simulink model "NCO_lfm_test"  (R2019b)
settings: Solver=FixedStepDiscrete  StartTime=0.0  StopTime=stoptime  RelTol=1e-3
InitFcn:
  | model_init
values from neighbouring files (symbols this model uses):
  chirp_dur_samp = fs*chirp_dur    (= 6400)    [model_init.m]
  end_inc = floor(f1*2^N / fs)    [model_init.m]
  start_inc = floor(f0*2^N / fs)    [model_init.m]
  Ts = 1/fs    (= 7.8125e-09)    [model_init.m]
libraries: hdlsllib x1, dsphdlsigops x1, dspsrcs4 x1
settings Model: DataTypeOverride=Off  Creator=tmealey  LastModifiedBy=ajtro
settings DataIOCC: SaveOutput=off  SignalLogging=off  DSMLogging=off  SaveTime=off  ReturnWorkspaceOutputs=off
settings OptimizationCC: BlockReduction=off  ConditionallyExecuteInputs=off  DefaultParameterBehavior=Inlined
settings DebuggingCC: AlgebraicLoopMsg=error  SingleTaskRateTransMsg=error
settings HardwareCC: ProdBitPerPointer=32  ProdBitPerSizeT=32  ProdBitPerPtrDiffT=32  ProdLargestAtomicFloat=None  ProdIntDivRoundTo=Undefined  ProdEndianess=Unspecified  ProdWordSize=32  ProdHWDeviceType=ASIC/FPGA->ASIC/FPGA  TargetBitPerPointer=64  TargetBitPerSizeT=64  TargetBitPerPtrDiffT=64  TargetLongLongMode=on  TargetIntDivRoundTo=Zero  TargetEndianess=LittleEndian  TargetWordSize=64  TargetHWDeviceType=Custom Processor->MATLAB Host Computer  ProdEqTarget=off

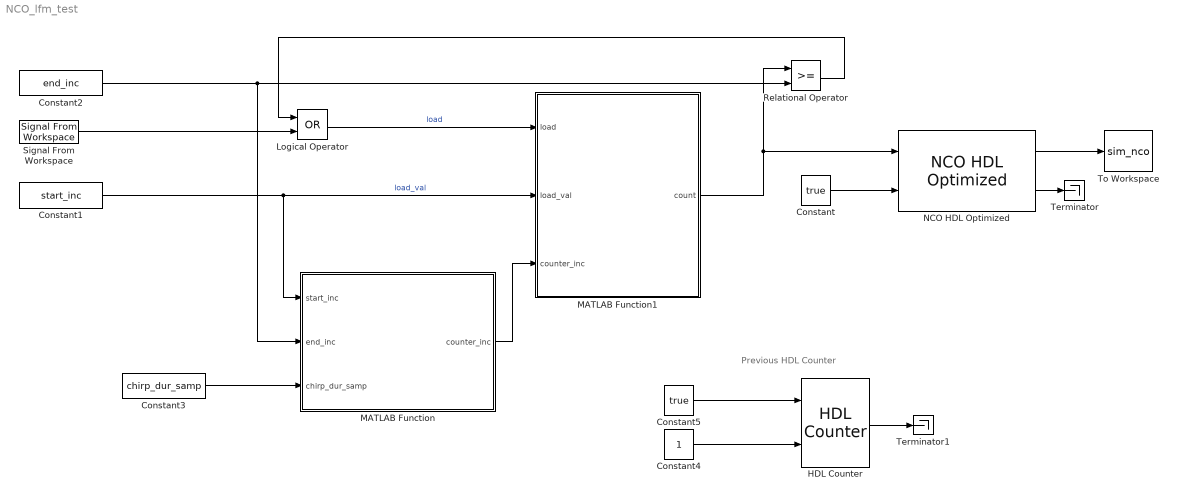
== system NCO_lfm_test ==
  note: Previous HDL Counter
  Constant : Constant  Value=true  SampleTime=-1
  Constant1 : Constant  Value=start_inc  OutDataTypeStr=uint16  SampleTime=Ts
  Constant2 : Constant  Value=end_inc  OutDataTypeStr=uint16  SampleTime=Ts
  Constant3 : Constant  Value=chirp_dur_samp  OutDataTypeStr=uint16  SampleTime=Ts
  Constant4 : Constant  OutDataTypeStr=uint16
  Constant5 : Constant  Value=true  SampleTime=-1
  HDL Counter : hdlsllib/Sources/HDL Counter  CountType=Free running  CountInit=0  CountStep=counter_inc  CountMax=end_inc  CountFromType=Initial value  CountFrom=0  CountResetPort=off  CountLoadPort=on  CountEnbPort=off  CountDirPort=off  CountDataType=Unsigned  CountWordLen=N  CountFracLen=0  CountSampTime=1
      settings: SourceProductName=Simulink
  Logical Operator : Logic  Operator=OR  AllPortsSameDT=off  OutDataTypeStr=boolean
  MATLAB Function : MATLAB Function  TreatAsAtomicUnit=on
  MATLAB Function1 : MATLAB Function  TreatAsAtomicUnit=on
  NCO HDL Optimized : dsphdlsigops/NCO HDL Optimized  PhaseIncrementSource=Input port  PhaseIncrement=100  PhaseOffsetSource=Property  PhaseOffset=0  DitherSource=Property  NumDitherBits=4  PhaseQuantization=on  NumQuantizerAccumulatorBits=12  LUTCompress=off  ResetAction=off  ValidInputPort=on  Waveform=Sine  PhasePort=off  SimulateUsing=Code generation  AccumulatorWL=N  OutputDataType=Binary point scaling  OutputWL=16  OutputFL=14
      settings: SourceProductName=DSP System Toolbox  SourceProductBaseCode=DS
  Relational Operator : RelationalOperator  OutDataTypeStr=boolean  RndMeth=Simplest
  Signal From Workspace : dspsrcs4/Signal From Workspace  X=true  Ts=Ts  nsamps=1  OutputAfterFinalValue=Setting to zero  ignoreOrWarnInputAndFrameLengths=off  OutputFrames=off
  Terminator : Terminator
  Terminator1 : Terminator
  To Workspace : ToWorkspace  VariableName=sim_nco  SampleTime=-1
      settings: Save2DSignal=2-D array (concatenate along first dimension)
  wires:
  MATLAB Function1/1(count) -> Relational Operator/1, NCO HDL Optimized/1
  Constant/1 -> NCO HDL Optimized/2
  NCO HDL Optimized/1 -> To Workspace/1
  NCO HDL Optimized/2 -> Terminator/1
  Logical Operator/1 -> MATLAB Function1/1(load)  "load"
  Relational Operator/1 -> Logical Operator/1
  Signal From Workspace/1 -> Logical Operator/2
  Constant2/1 -> MATLAB Function/2(end_inc), Relational Operator/2
  Constant3/1 -> MATLAB Function/3(chirp_dur_samp)
  MATLAB Function/1(counter_inc) -> MATLAB Function1/3(counter_inc)
  Constant4/1 -> HDL Counter/2
  Constant5/1 -> HDL Counter/1
  HDL Counter/1 -> Terminator1/1
  Constant1/1 -> MATLAB Function/1(start_inc), MATLAB Function1/2(load_val)  "load_val"

== matlab function NCO_lfm_test/MATLAB Function1 ==
  data: load input; count output; load_val input; counter_inc input
function count = chirp_Counter(load, load_val, counter_inc)
%#codegen
% Counter that allows counter_increment to change 
% on the fly
% Inputs:
% boolean - load
% uint16  - load_val
% uint16  - counter_inc

% Initialize count_register
persistent count_register;
if isempty(count_register) % initialize from example
% if ~exist('count_register','var') % My usual way to initialize
   count_register = 0; 
end


if(load == true)
    count_register = load_val;    
else
    count_register = counter_inc + count_register;
end

count = count_register;

== matlab function NCO_lfm_test/MATLAB Function ==
  data: start_inc input; counter_inc output; end_inc input; chirp_dur_samp input
function counter_inc = calculate_chirp_increment(start_inc, end_inc, chirp_dur_samp)
N = 16;
fs = 128e6;
Ts = 1/fs;
f0 = 0e6;
f1 = 25e6;

chirp_dur = 50e-6;

chirp_dur_samp = fs*chirp_dur;

start_inc = floor(f0*2^N / fs);
end_inc = floor(f1*2^N / fs);

counter_inc = (end_inc-start_inc)/chirp_dur_samp;

% stoptime = chirp_dur;
